simulink model "a3"  (R2023b)
settings: Solver=VariableStepAuto  StartTime=0.0  StopTime=50.0  RelTol=1e-3
values from neighbouring files (symbols this model uses):
  C = [0 57.3 0 0 0;0 0 0 1 0;0.0208 15.2 0 1.45 0]    [f16model.m]
  dt = 50/1000    (= 0.05)    [f16model.m]
  K_int = K(:,end)    [f16model.m]
  K_noint = K(:,1:end-1)    [f16model.m]
libraries: cstblocks x35, simulink x9
settings Model: Creator=valter  LastModifiedBy=valter

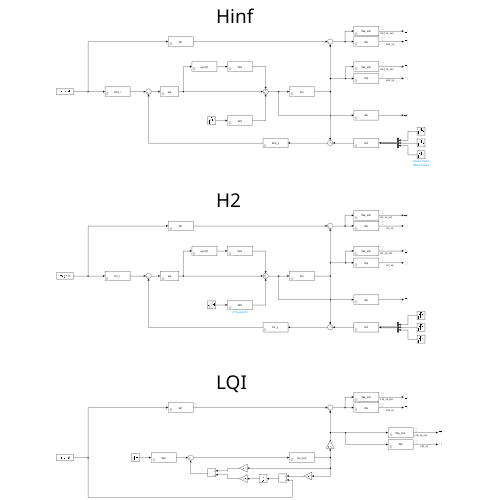
[thumbnail: Simulink's stored preview of the top-level diagram]
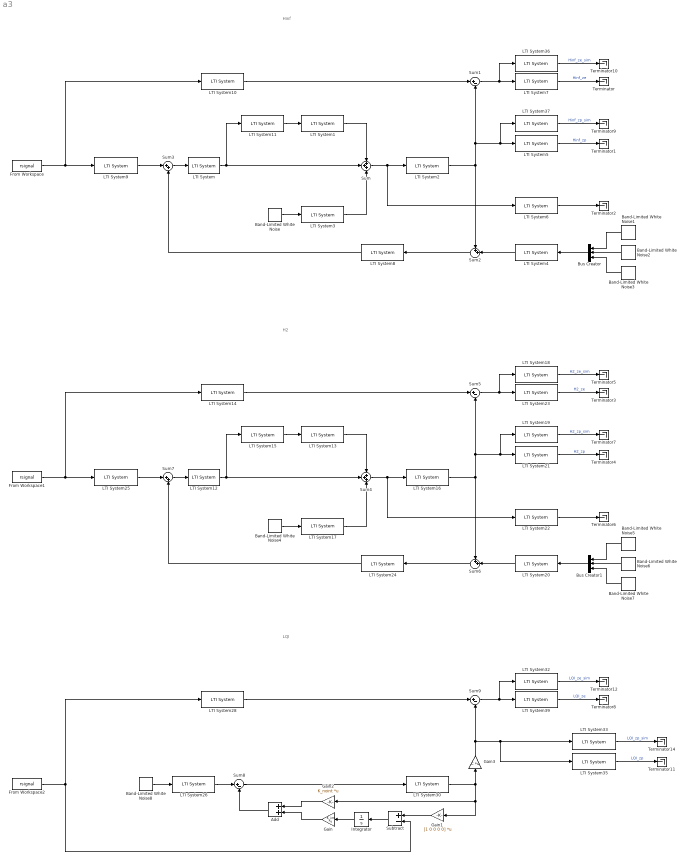
== system a3 ==
  note: Hinf
  note: H2
  note: LQI
  Add : Sum
  Band-Limited White Noise{,1..8} (9 alike) : simulink/Sources/Band-Limited White Noise  Cov=1  Ts=dt  seed=[23341]
  Bus Creator : BusCreator  Inputs=3
  Bus Creator1 : BusCreator  Inputs=3
  From Workspace : FromWorkspace  VariableName=rsignal  SampleTime=dt
  From Workspace1 : FromWorkspace  VariableName=rsignal  SampleTime=dt
  From Workspace2 : FromWorkspace  VariableName=rsignal  SampleTime=dt
  Gain : Gain  Gain=K_int  Multiplication=Matrix(K*u)
  Gain1 : Gain  Gain=[1 0 0 0 0]  Multiplication=Matrix(K*u)
  Gain2 : Gain  Gain=K_noint  Multiplication=Matrix(K*u)
  Gain3 : Gain  Gain=C  Multiplication=Matrix(K*u)
  Integrator : Integrator
  LTI System : cstblocks/LTI System  sys=Ga  IC=[]  PadeOrder=0
  LTI System1 : cstblocks/LTI System  sys=Wm  IC=[]  PadeOrder=0
  LTI System10 : cstblocks/LTI System  sys=Wr  IC=[]  PadeOrder=0
  LTI System11 : cstblocks/LTI System  sys=eye(2)  IC=[]  PadeOrder=0
  LTI System12 : cstblocks/LTI System  sys=Ga  IC=[]  PadeOrder=0
  LTI System13 : cstblocks/LTI System  sys=Wm  IC=[]  PadeOrder=0
  LTI System14 : cstblocks/LTI System  sys=Wr  IC=[]  PadeOrder=0
  LTI System15 : cstblocks/LTI System  sys=eye(2)  IC=[]  PadeOrder=0
  LTI System16 : cstblocks/LTI System  sys=Gn  IC=[]  PadeOrder=0
  LTI System17 : cstblocks/LTI System  sys=Wd  IC=[]  PadeOrder=0
  LTI System18 : cstblocks/LTI System  sys=We_sim  IC=[]  PadeOrder=0
  LTI System19 : cstblocks/LTI System  sys=Wp_sim  IC=[]  PadeOrder=0
  LTI System2 : cstblocks/LTI System  sys=Gn  IC=[]  PadeOrder=0
  LTI System20 : cstblocks/LTI System  sys=Wn  IC=[]  PadeOrder=0
  LTI System21 : cstblocks/LTI System  sys=Wp  IC=[]  PadeOrder=0
  LTI System22 : cstblocks/LTI System  sys=Wu  IC=[]  PadeOrder=0
  LTI System23 : cstblocks/LTI System  sys=We  IC=[]  PadeOrder=0
  LTI System24 : cstblocks/LTI System  sys=K2_y  IC=[]  PadeOrder=0
  LTI System25 : cstblocks/LTI System  sys=K2_r  IC=[]  PadeOrder=0
  LTI System26 : cstblocks/LTI System  sys=Wd  IC=[]  PadeOrder=0
  LTI System28 : cstblocks/LTI System  sys=Wr  IC=[]  PadeOrder=0
  LTI System3 : cstblocks/LTI System  sys=Wd  IC=[]  PadeOrder=0
  LTI System30 : cstblocks/LTI System  sys=Gn_sim  IC=[]  PadeOrder=0
  LTI System32 : cstblocks/LTI System  sys=We_sim  IC=[]  PadeOrder=0
  LTI System33 : cstblocks/LTI System  sys=Wp_sim  IC=[]  PadeOrder=0
  LTI System35 : cstblocks/LTI System  sys=Wp  IC=[]  PadeOrder=0
  LTI System36 : cstblocks/LTI System  sys=We_sim  IC=[]  PadeOrder=0
  LTI System37 : cstblocks/LTI System  sys=Wp_sim  IC=[]  PadeOrder=0
  LTI System39 : cstblocks/LTI System  sys=We  IC=[]  PadeOrder=0
  LTI System4 : cstblocks/LTI System  sys=Wn  IC=[]  PadeOrder=0
  LTI System5 : cstblocks/LTI System  sys=Wp  IC=[]  PadeOrder=0
  LTI System6 : cstblocks/LTI System  sys=Wu  IC=[]  PadeOrder=0
  LTI System7 : cstblocks/LTI System  sys=We  IC=[]  PadeOrder=0
  LTI System8 : cstblocks/LTI System  sys=Kinf_y  IC=[]  PadeOrder=0
  LTI System9 : cstblocks/LTI System  sys=Kinf_r  IC=[]  PadeOrder=0
  Subtract : Sum  Inputs=+-
  Sum : Sum  Inputs=+++
  Sum{1,5,8..9} (4 alike) : Sum  Inputs=|+-
  Sum2 : Sum  Inputs=++|
  Sum3 : Sum  Inputs=|++
  Sum4 : Sum  Inputs=+++
  Sum6 : Sum  Inputs=++|
  Sum7 : Sum  Inputs=|++
  Terminator{,1..12,14} (14 alike) : Terminator
  wires:
  From Workspace/1 -> LTI System10/1, LTI System9/1
  LTI System/1 -> LTI System11/1, Sum/2
  LTI System1/1 -> Sum/1
  LTI System3/1 -> Sum/3
  Sum/1 -> LTI System6/1, LTI System2/1
  LTI System2/1 -> Sum2/1, LTI System37/1, LTI System5/1, Sum1/2
  Band-Limited White Noise/1 -> LTI System3/1
  LTI System4/1 -> Sum2/2
  LTI System9/1 -> Sum3/1
  Sum3/1 -> LTI System/1
  LTI System7/1 -> Terminator/1  "Hinf_ze"
  LTI System6/1 -> Terminator2/1
  LTI System5/1 -> Terminator1/1  "Hinf_zp"
  LTI System8/1 -> Sum3/2
  Sum2/1 -> LTI System8/1
  Sum1/1 -> LTI System36/1, LTI System7/1
  LTI System10/1 -> Sum1/1
  LTI System11/1 -> LTI System1/1
  Bus Creator/1 -> LTI System4/1
  Band-Limited White Noise2/1 -> Bus Creator/2
  Band-Limited White Noise1/1 -> Bus Creator/1
  Band-Limited White Noise3/1 -> Bus Creator/3
  LTI System36/1 -> Terminator10/1  "Hinf_ze_sim"
  LTI System37/1 -> Terminator9/1  "Hinf_zp_sim"
  LTI System13/1 -> Sum4/1
  LTI System17/1 -> Sum4/3
  From Workspace1/1 -> LTI System14/1, LTI System25/1
  LTI System22/1 -> Terminator6/1
  LTI System20/1 -> Sum6/2
  LTI System23/1 -> Terminator3/1  "H2_ze"
  Sum4/1 -> LTI System22/1, LTI System16/1
  Band-Limited White Noise4/1 -> LTI System17/1
  LTI System19/1 -> Terminator7/1  "H2_zp_sim"
  LTI System12/1 -> LTI System15/1, Sum4/2
  Band-Limited White Noise5/1 -> Bus Creator1/1
  Bus Creator1/1 -> LTI System20/1
  Band-Limited White Noise6/1 -> Bus Creator1/2
  LTI System14/1 -> Sum5/1
  LTI System24/1 -> Sum7/2
  LTI System21/1 -> Terminator4/1  "H2_zp"
  Sum6/1 -> LTI System24/1
  LTI System15/1 -> LTI System13/1
  Sum5/1 -> LTI System18/1, LTI System23/1
  Band-Limited White Noise7/1 -> Bus Creator1/3
  LTI System16/1 -> Sum6/1, LTI System19/1, LTI System21/1, Sum5/2
  LTI System25/1 -> Sum7/1
  Sum7/1 -> LTI System12/1
  LTI System18/1 -> Terminator5/1  "H2_ze_sim"
  From Workspace2/1 -> Subtract/2, LTI System28/1
  LTI System39/1 -> Terminator8/1  "LQI_ze"
  LTI System33/1 -> Terminator14/1  "LQI_zp_sim"
  LTI System28/1 -> Sum9/1
  LTI System35/1 -> Terminator11/1  "LQI_zp"
  Sum9/1 -> LTI System32/1, LTI System39/1
  LTI System30/1 -> Gain1/1, Gain2/1, Gain3/1
  LTI System32/1 -> Terminator12/1  "LQI_ze_sim"
  Gain1/1 -> Subtract/1
  Subtract/1 -> Integrator/1
  Integrator/1 -> Gain/1
  Band-Limited White Noise8/1 -> LTI System26/1
  LTI System26/1 -> Sum8/1
  Sum8/1 -> LTI System30/1
  Gain2/1 -> Add/1
  Gain/1 -> Add/2
  Add/1 -> Sum8/2
  Gain3/1 -> LTI System35/1, LTI System33/1, Sum9/2
